simulink model "single_phase_inverter"  (R2021a)
settings: Solver=VariableStepAuto  StartTime=0.0  StopTime=0.04  RelTol=1e-3  EnableMultiTasking=on
libraries: spsIGBTDiodeLib x8, spsSeriesRLCBranchLib x2, spsDCVoltageSourceLib x2, spsTriangleGeneratorLib x2, spsVoltageMeasurementLib x2, spspowerguiLib x1
settings Model: Creator=Srinivasan  LastModifiedBy=SK
settings SolverCC: AlgebraicLoopSolver=TrustRegion
settings DataIOCC: ReturnWorkspaceOutputs=off
settings OptimizationCC: LifeSpan=inf
settings DebuggingCC: SFUnexpectedBacktrackingDiag=warning  SFNoUnconditionalDefaultTransitionDiag=warning  SFMachineParentedDataDiag=warning  ArithmeticOperatorsInVariantConditions=warning
settings SFSimCC: SimUseLocalCustomCode=off  CustomCodeUndefinedFunction=UseInterfaceOnly
settings RTWCC: RTWUseLocalCustomCode=off
settings CodeAppCC: StateflowObjectComments=on
settings GRTTargetCC: TargetLangStandard=C89/C90 (ANSI)
settings ConfigComp: CovMetricSettings=dw  CovSaveCumulativeToWorkspaceVar=on  CovSaveSingleToWorkspaceVar=on  CovExternalEMLEnable=off
settings SimscapeCC: SimscapeNormalizeSystem=off

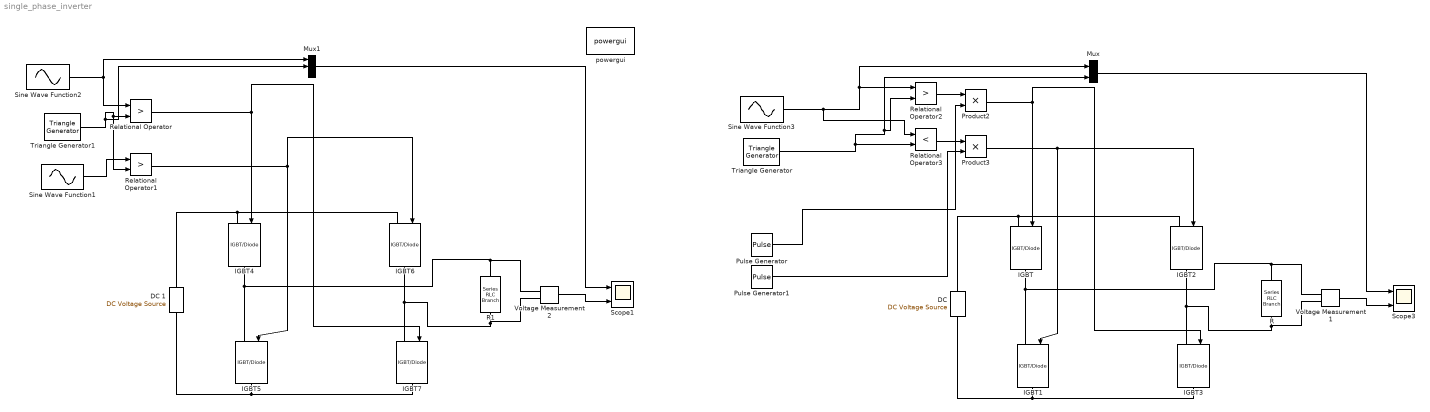
== system single_phase_inverter ==
  " R" : spsSeriesRLCBranchLib/Series RLC Branch  LConnTagsString=__new0  RConnTagsString=__new0  BranchType=R  Resistance=10  Inductance=0.1  SetiL0=off  InitialCurrent=0  Capacitance=0  Setx0=off  InitialVoltage=0  Measurements=None
  " R1" : spsSeriesRLCBranchLib/Series RLC Branch  LConnTagsString=__new0  RConnTagsString=__new0  BranchType=R  Resistance=10  Inductance=0.1  SetiL0=off  InitialCurrent=0  Capacitance=0  Setx0=off  InitialVoltage=0  Measurements=None
  "DC " : spsDCVoltageSourceLib/DC Voltage Source  Amplitude=24  Measurements=None
  DC 1 : spsDCVoltageSourceLib/DC Voltage Source  Amplitude=24  Measurements=None
  IGBT{,1..7} (8 alike) : spsIGBTDiodeLib/IGBT//Diode  Ron=1e-3  Rs=1e5  Cs=inf  Measurements=off
  Mux : Mux  Inputs=2
  Mux1 : Mux  Inputs=3
  Product2 : Product
  Product3 : Product
  Pulse Generator : DiscretePulseGenerator  PulseType=Time based  Period=0.02  PulseWidth=50
  Pulse Generator1 : DiscretePulseGenerator  PulseType=Time based  Period=0.02  PulseWidth=50  PhaseDelay=0.01
  Relational Operator : RelationalOperator  Operator=>  OutDataTypeStr=boolean  RndMeth=Simplest
  Relational Operator1 : RelationalOperator  Operator=>  OutDataTypeStr=boolean  RndMeth=Simplest
  Relational Operator2 : RelationalOperator  Operator=>  OutDataTypeStr=boolean  RndMeth=Simplest
  Relational Operator3 : RelationalOperator  Operator=<  OutDataTypeStr=boolean  RndMeth=Simplest
  Scope1 : Scope  NumInputPorts=2
  Scope3 : Scope  NumInputPorts=2
  Sine Wave Function1 : Sin  Frequency=2*pi*50  Phase=pi  SampleTime=0
  Sine Wave Function2 : Sin  Frequency=2*pi*50  SampleTime=0
  Sine Wave Function3 : Sin  Frequency=2*pi*50  SampleTime=0
  Triangle Generator : spsTriangleGeneratorLib/Triangle Generator  Freq=1e3  Phase=90  Ts=0
  Triangle Generator1 : spsTriangleGeneratorLib/Triangle Generator  Freq=1e3  Phase=90  Ts=0
  Voltage Measurement1 : spsVoltageMeasurementLib/Voltage Measurement  PhasorSimulation=off  OutputType=Complex  PSBequivalent=0
  Voltage Measurement2 : spsVoltageMeasurementLib/Voltage Measurement  PhasorSimulation=off  OutputType=Complex  PSBequivalent=0
  powergui : spspowerguiLib/powergui  Priority=1  SimulationMode=Discrete  SampleTime=50e-6  frequency=60  Iterations=50  frequencyindice=0  Pbase=100e6  ErrMax=1e-4  UnitsV=kV  UnitsW=MW  buscounter=0  FunctionMessages=off  echomessages=off  EnableUseOfTLC=off  CurrentSourceSwitches=off  DisableSnubberDevices=off  DisableRonSwitches=off  DisableVfSwitches=off  DisplayEquations=off  AutomaticDiscreteSolvers=off  SolverType=Tustin/Backward Euler (TBE)  Interpol=off  ExternalGateDelay=off  methode=off  Ts=10  x0status=blocks  SPID=off  SwTol=0  HookPort=off  NonlinearTolerance=1e-4  nMaxIteration=100  ContinueOnMaxIteration=off  RestoreLinks=warning  ResistiveCurrentMeasurement=off  Frange=[0:2:500]  Ylog=off  Xlog=on  ShowGrid=off  save=off  variable=ZData  structure=0  ZoomFFT=off  StartTime=0.0  cycles=1  DisplayStyle=1  fundamental=60  FreqAxis=off  MaxFrequency=1000  frequencyindicesteady=1  RmsSteady=1  display=off
  wires:
  Voltage Measurement1/1 -> Scope3/2
  Mux/1 -> Scope3/1
  Triangle Generator/1 -> Relational Operator2/2, Mux/2, Relational Operator3/2
  Product2/1 -> IGBT3/1, IGBT/1
  Mux1/1 -> Scope1/1
  Voltage Measurement2/1 -> Scope1/2
  Triangle Generator1/1 -> Mux1/2, Relational Operator1/2, Relational Operator/2
  Relational Operator1/1 -> IGBT6/1, IGBT5/1
  Sine Wave Function2/1 -> Mux1/1, Relational Operator/1
  Relational Operator/1 -> IGBT7/1, IGBT4/1
  Sine Wave Function1/1 -> Relational Operator1/1
  Sine Wave Function3/1 -> Relational Operator3/1, Relational Operator2/1, Mux/1
  Pulse Generator/1 -> Product2/2
  Relational Operator2/1 -> Product2/1
  Relational Operator3/1 -> Product3/1
  Product3/1 -> IGBT1/1, IGBT2/1
  Pulse Generator1/1 -> Product3/2
  connections:
  IGBT/RConn1 -- Voltage Measurement1/LConn1 -- " R"/LConn1 -- IGBT1/LConn1
  IGBT3/LConn1 -- Voltage Measurement1/LConn2 -- " R"/RConn1 -- IGBT2/RConn1
  IGBT2/LConn1 -- "DC "/RConn1 -- IGBT/LConn1
  IGBT1/RConn1 -- "DC "/LConn1 -- IGBT3/RConn1
  " R1"/LConn1 -- IGBT4/RConn1 -- IGBT5/LConn1 -- Voltage Measurement2/LConn1
  IGBT7/RConn1 -- IGBT5/RConn1 -- DC 1/LConn1
  IGBT6/RConn1 -- IGBT7/LConn1 -- Voltage Measurement2/LConn2 -- " R1"/RConn1
  IGBT4/LConn1 -- IGBT6/LConn1 -- DC 1/RConn1
